simulink model "FOC_Motor_Control"  (R2020b)
settings: Solver=FixedStepAuto  StartTime=0.0  StopTime=10.0  FixedStep=Fixed_Step_Size  RelTol=1e-3
values from neighbouring files (symbols this model uses):
  Angle = 1.0    [Hall_FOC_Data.sldd]
  Angle_offset = 0.1985    [Hall_FOC_Data.sldd]
  atan_table = -1.5690511 -1.5690503 -1.5690495 -1.5690485 -1.5690477 -1.5690469 -1.569046 -1.5690452 -1.5690442 -1.5690434 -1.5690426 -1.5690417 -1.5690409 -1.5690399 -1.5690391 -1.5690383 -1.5690374 -1.5690365 -1.5690356 -1.5690348 -1.5690339 -1.569033 -1.5690322 -1.5690314 -1.5690304 -1.5690296 -1.5690287 -1.5690278 -1.5690269 -1.5690261 -1.5690252 -1.5690243 -1.5690234 -1.5690225 -1.5690217 -1.5690207 -1.569    [Hall_FOC_Data.sldd]
  Cosine_table = 1.0 0.99999529 0.99999058 0.99998587 0.99998116 0.99996704 0.99995291 0.99993885 0.99992472 0.99990118 0.99987763 0.99985409 0.9998306 0.99979764 0.99976468 0.99973178 0.99969882 0.99965644 0.99961412 0.99957174 0.99952942 0.99947762 0.99942589 0.99937415 0.99932235 0.9992612 0.99920005 0.99913889 0.99907768 0.99900717 0.99893659 0.99886602 0.99879545 0.99871546 0.99863547 0.99855554 0.99847555 0.    [Hall_FOC_Data.sldd]
  Dead_Com_Enable = 0.0    [Hall_FOC_Data.sldd]
  Dead_Time = 0.0    [Hall_FOC_Data.sldd]
  FF_Enable = 0.0    [Hall_FOC_Data.sldd]
  Flux = 0.0260812    [Hall_FOC_Data.sldd]
  FluxWeak_Enable = 0.0    [Hall_FOC_Data.sldd]
  FluxWeak_Idref_max = 0.0    [Hall_FOC_Data.sldd]
  FluxWeak_Idref_min = -200.0    [Hall_FOC_Data.sldd]
  FluxWeak_Ki = 50.0    [Hall_FOC_Data.sldd]
  FluxWeak_Kp = 1.2    [Hall_FOC_Data.sldd]
  HaLL_AngleShift = -0.25    [Hall_FOC_Data.sldd]
  HaLL_Sector1 = 5.236    [Hall_FOC_Data.sldd]
  HaLL_Sector2 = 1.0472    [Hall_FOC_Data.sldd]
  HaLL_Sector3 = 0.0    [Hall_FOC_Data.sldd]
  HaLL_Sector4 = 3.1415    [Hall_FOC_Data.sldd]
  HaLL_Sector5 = 4.1888    [Hall_FOC_Data.sldd]
  HaLL_Sector6 = 2.0944    [Hall_FOC_Data.sldd]
  HaLL_Timer_T = 1.0E-5    [Hall_FOC_Data.sldd]
  Harmonic_Com_Enable = 0.0    [Hall_FOC_Data.sldd]
  Harmonic_Id5th_Ki = 32.0    [Hall_FOC_Data.sldd]
  Harmonic_Id5th_Kp = 1.2    [Hall_FOC_Data.sldd]
  Harmonic_Id5th_Max = 60.0    [Hall_FOC_Data.sldd]
  Harmonic_Id5th_Min = -60.0    [Hall_FOC_Data.sldd]
  Harmonic_Id7th_Ki = 24.0    [Hall_FOC_Data.sldd]
  Harmonic_Id7th_Kp = 0.8    [Hall_FOC_Data.sldd]
  Harmonic_Id7th_Max = 60.0    [Hall_FOC_Data.sldd]
  Harmonic_Id7th_Min = -60.0    [Hall_FOC_Data.sldd]
  Harmonic_Iq5th_Ki = 32.0    [Hall_FOC_Data.sldd]
  Harmonic_Iq5th_Kp = 1.2    [Hall_FOC_Data.sldd]
  Harmonic_Iq5th_Max = 60.0    [Hall_FOC_Data.sldd]
  Harmonic_Iq5th_Min = -60.0    [Hall_FOC_Data.sldd]
  Harmonic_Iq7th_Ki = 24.0    [Hall_FOC_Data.sldd]
  Harmonic_Iq7th_Kp = 0.8    [Hall_FOC_Data.sldd]
  Harmonic_Iq7th_Max = 60.0    [Hall_FOC_Data.sldd]
  Harmonic_Iq7th_Min = -60.0    [Hall_FOC_Data.sldd]
  ID_Ki = 0.8    [Hall_FOC_Data.sldd]
  ID_Kp = 3.2    [Hall_FOC_Data.sldd]
  IQ_Ki = 0.32    [Hall_FOC_Data.sldd]
  IQ_Kp = 3.3    [Hall_FOC_Data.sldd]
  LADRC_b0 = 80000.0    [Hall_FOC_Data.sldd]
  LADRC_Omega_c = 80.0    [Hall_FOC_Data.sldd]
  Ld = 0.004    [Hall_FOC_Data.sldd]
  Lq = 0.0042    [Hall_FOC_Data.sldd]
  MTPA_id_table = 0.22889 0.23462678 0.23770036 0.2381243 0.23591207 0.23107713 0.2236329 0.21359272 0.20096992 0.18577772 0.16802935 0.14773798 0.12491672 0.099578641 0.071736768 0.041404068 0.0085934745 -0.026682133 -0.064409919 -0.10457709 -0.14717092 -0.1921787 -0.2395878 -0.28938559 -0.34155953 -0.39609709 -0.45298585 -0.51221335 -0.57376724 -0.63763517 -0.70380485 -0.77226412 -0.84300071 -0.91600245 -0.991257    [Hall_FOC_Data.sldd]
  MTPA_iq_table = -1.0417 -0.16083497 0.71926296 1.5985928 2.4771533 3.3549435 4.2319627 5.1082091 5.9836826 6.8583813 7.732305 8.6054525 9.4778223 10.349415 11.220228 12.090261 12.959513 13.827983 14.69567 15.562573 16.428694 17.294027 18.158575 19.022335 19.885307 20.747492 21.608887 22.469492 23.329306 24.188328 25.046556 25.903992 26.760633 27.616482 28.471533 29.325788 30.179247 31.031908 31.883772 32.734837 3    [Hall_FOC_Data.sldd]
  MTPA_Te_Max = 800.0    [Hall_FOC_Data.sldd]
  MTPA_Te_Min = 0.0    [Hall_FOC_Data.sldd]
  Over_modulation = 0.0    [Hall_FOC_Data.sldd]
  Pole_Pairs = 2.0    [Hall_FOC_Data.sldd]
  PWM_Frequency = 10000.0    [Hall_FOC_Data.sldd]
  R = 0.4    [Hall_FOC_Data.sldd]
  Sine_table = 0.0 0.0015339879 0.0030679768 0.0046019657 0.0061359555 0.0076698866 0.0092038177 0.010737749 0.012271681 0.013805497 0.015339312 0.016873131 0.018406944 0.019940587 0.021474229 0.023007872 0.024541514 0.026074925 0.027608337 0.029141748 0.03067516 0.032208283 0.033741407 0.035274528 0.036807653 0.038340431 0.039873205 0.04140598 0.042938754 0.04447113 0.046003502 0.047535874 0.049068246 0.0506001    [Hall_FOC_Data.sldd]
  Speed_Ki = 0.633    [Hall_FOC_Data.sldd]
  Speed_Kp = 0.0267    [Hall_FOC_Data.sldd]
  Speed_PI_OutputMax = 5.0    [Hall_FOC_Data.sldd]
  Speed_PI_OutputMin = -5.0    [Hall_FOC_Data.sldd]
  SpeedFilter_Fn = 0.2    [Hall_FOC_Data.sldd]
  TorqueMode = 0.0    [Hall_FOC_Data.sldd]
undefined symbols (not defined in the file or in its folder): DiscIntNeverNeededParam, inverter, magnitude, SVPWM
libraries: simulink x6, powerlib_extras x4, pid_lib x1
(part 2 of 5)

== system FOC_Motor_Control/Motor_Control/Motor_Control_Function/SYM_State_10ms/LPF1 ==
  u : Inport
  Add : Sum  Inputs=+-
  Add1 : Sum
  Constant1 : Constant  Value=0.005  OutDataTypeStr=single
  Divide1 : Product  Inputs=**
  Unit Delay : UnitDelay  SampleTime=-1  HasFrameUpgradeWarning=on
  y : Outport
  wires:
  Constant1/1 -> Divide1/1
  u/1 -> Add/1
  Add/1 -> Divide1/2
  Divide1/1 -> Add1/1
  Unit Delay/1 -> Add/2, Add1/2
  Add1/1 -> Unit Delay/1, y/1

== system FOC_Motor_Control/Motor_Control/Motor_Control_Function/SYM_State_10ms/Power_Cacl ==
  Id : Inport
  Vd : Inport  Port=2
  Iq : Inport  Port=3
  Vq : Inport  Port=4
  Add : Sum
  Product : Product
  Product1 : Product
  Power : Outport
  wires:
  Id/1 -> Product/1
  Vd/1 -> Product/2
  Iq/1 -> Product1/1
  Vq/1 -> Product1/2
  Product/1 -> Add/1
  Product1/1 -> Add/2
  Add/1 -> Power/1

== system FOC_Motor_Control/Motor_Control/Motor_Control_Function/SYM_State_10ms/Torque_Cacl ==
  Id : Inport
  Iq : Inport  Port=2
  Constant : Constant  Value=3/2  OutDataTypeStr=single
  Constant1 : Constant  Value=Pole_Pairs  OutDataTypeStr=single
  Constant2 : Constant  Value=Flux  OutDataTypeStr=single
  Constant3 : Constant  Value=Ld  OutDataTypeStr=single
  Constant4 : Constant  Value=Lq  OutDataTypeStr=single
  Product{,1..4} (5 alike) : Product
  Subtract : Sum
  Subtract1 : Sum  Inputs=+-
  Torque : Outport
  wires:
  Constant1/1 -> Product/1
  Constant/1 -> Product/2
  Constant2/1 -> Product1/1
  Iq/1 -> Product1/2, Product3/1
  Product1/1 -> Subtract/1
  Constant3/1 -> Subtract1/1
  Constant4/1 -> Subtract1/2
  Subtract1/1 -> Product2/1
  Id/1 -> Product2/2
  Product2/1 -> Product3/2
  Product3/1 -> Subtract/2
  Product/1 -> Product4/1
  Subtract/1 -> Product4/2
  Product4/1 -> Torque/1

== system FOC_Motor_Control/Motor_Control/Motor_Control_Function/Angle_Speed_100us/Resolver_Observer/Angle_calibration ==
  Angle_input : Inport
  Angle_offset : Constant  Value=Angle_offset
  If Action Subsystem1 : Subsystem  TreatAsAtomicUnit=on
  If Action Subsystem2 : Subsystem  TreatAsAtomicUnit=on
  If1 : If  IfExpression=u1 > 6.283185307
  Merge1 : Merge
  Subtract1 : Sum
  Angle_output : Outport
  wires:
  Angle_input/1 -> Subtract1/1
  Merge1/1 -> Angle_output/1
  Angle_offset/1 -> Subtract1/2  "Control_ModeCommand"
  If1/1 -> If Action Subsystem2/Action
  If1/2 -> If Action Subsystem1/Action
  If Action Subsystem2/1(Out1) -> Merge1/1
  Subtract1/1 -> If Action Subsystem1/1(In1), If Action Subsystem2/1(In1), If1/1
  If Action Subsystem1/1(Out1) -> Merge1/2

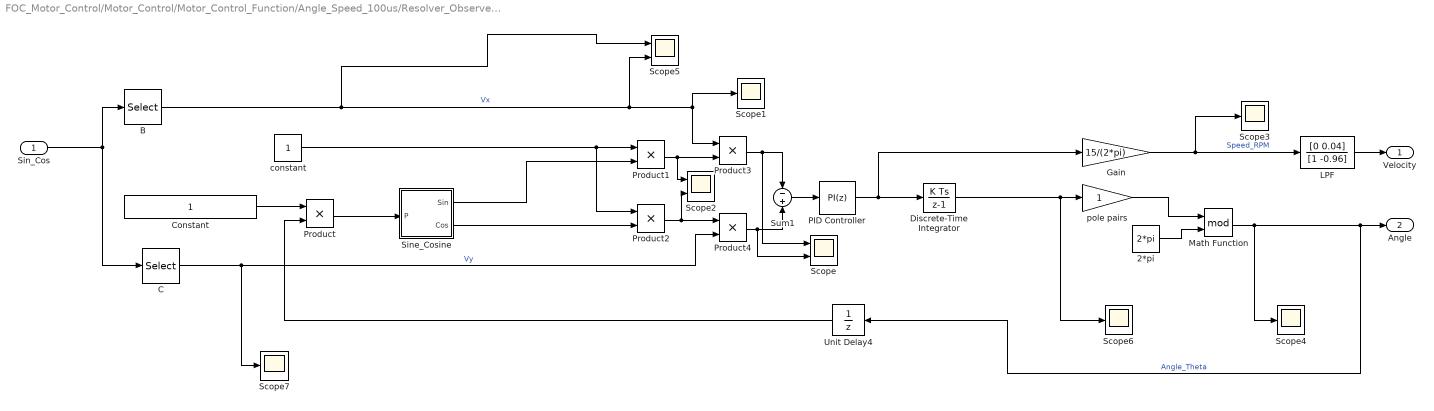
== system FOC_Motor_Control/Motor_Control/Motor_Control_Function/Angle_Speed_100us/Resolver_Observer/Resolver_Angle_cacl ==
  Sin_Cos : Inport
  2*pi : Constant  Value=2*pi  OutDataTypeStr=single  SampleTime=-1
  B : Selector  IndexMode=Zero-based  InputPortWidth=2  IndexOptions=Index vector (dialog)  Indices=0  OutputSizes=1
  C : Selector  IndexMode=Zero-based  InputPortWidth=2  IndexOptions=Index vector (dialog)  Indices=1  OutputSizes=1
  Constant : Constant  OutDataTypeStr=single  SampleTime=-1
  Discrete-Time Integrator : DiscreteIntegrator  SampleTime=-1  ICPrevOutput=DiscIntNeverNeededParam  ICPrevScaledInput=DiscIntNeverNeededParam
  Gain : Gain  Gain=15/(2*pi)
  LPF : DiscreteFilter  Numerator=[0 0.04]  Denominator=[1 -0.96]
  Math Function : Math  Operator=mod  SignedPower=on  SaturateOnIntegerOverflow=on
  PID Controller : pid_lib/PID Controller  Controller=PI  Form=Parallel  TimeDomain=Discrete-time  UseExternalTs=off  SampleTime=-1  IntegratorMethod=Forward Euler  FilterMethod=Forward Euler  ControllerParametersSource=internal  P=141  I=10000  D=0  UseFilter=off  N=100  TunerSelectOption=Transfer Function Based (PID Tuner App)  InitialConditionSource=internal  InitialConditionForIntegrator=0  InitialConditionForFilter=0  DifferentiatorICPrevScaledInput=0  ExternalReset=none  TrackingMode=off  Kt=1  LimitOutput=off  SatLimitsSource=internal  UpperSaturationLimit=inf  LowerSaturationLimit=-inf  LinearizeAsGain=on  AntiWindupMode=none  Kb=1  POutMin=[]  POutMax=[]  IOutMin=[]  IOutMax=[]  DOutMin=[]  DOutMax=[]  NOutMin=[]  NOutMax=[]  SumOutMin=[]  SumOutMax=[]  SaturationOutMin=[]  SaturationOutMax=[]  PParamMin=[]  PParamMax=[]  IParamMin=[]  IParamMax=[]  DParamMin=[]  DParamMax=[]  NParamMin=[]  NParamMax=[]  KbParamMin=[]  KbParamMax=[]  KtParamMin=[]  KtParamMax=[]  KbOutMin=[]  KbOutMax=[]  KtOutMin=[]  KtOutMax=[]  IntegratorOutMin=[]  IntegratorOutMax=[]  FilterOutMin=[]  FilterOutMax=[]  SumI1OutMin=[]  SumI1OutMax=[]  SumI2OutMin=[]  SumI2OutMax=[]  SumI3OutMin=[]  SumI3OutMax=[]  SumI4OutMin=[]  SumI4OutMax=[]  SumDOutMin=[]  SumDOutMax=[]  DifferentiatorOutMin=[]  DifferentiatorOutMax=[]  FilterDiffOutCoefMin=[]  FilterDiffOutCoefMax=[]  ReciprocalOutMin=[]  ReciprocalOutMax=[]  SumDenOutMin=[]  SumDenOutMax=[]  SumNumOutMin=[]  SumNumOutMax=[]  DivideOutMin=[]  DivideOutMax=[]  UdiffTsProdOutMin=[]  UdiffTsProdOutMax=[]  NTsProdOutMin=[]  NTsProdOutMax=[]  UintegralTsProdOutMin=[]  UintegralTsProdOutMax=[]  UngainTsProdOutMin=[]  UngainTsProdOutMax=[]  IntegratorContinuousStateAttributes=''  IntegratorStateMustResolveToSignalObject=off  IntegratorRTWStateStorageClass=Auto  FilterContinuousStateAttributes=''  FilterStateMustResolveToSignalObject=off  FilterRTWStateStorageClass=Auto  ParallelPVariant=InternalParameters  IdealPVariant=Disabled  IVariant=InternalParameters  DVariant=Disabled  IntegratorVariant=Discrete  SatVariant=Disabled  AWVariant=Passthrough  PCopyVariant=Disabled  TRVariant=Disabled  FdbkBlocksVariant=Forward  IdealPFdbkVariant=Disabled  SatFdbkVariant=Disabled  DerivativeFilterVariant=Disabled  NVariant=Disabled  NCopyVariant=Disabled_SignalSpec  FilterICVariant=Disabled  IntegratorICVariant=InternalICs  ExternalResetVariant=Disabled  TRSumVariant=Passthrough  SumFdbkVariant=Disabled  SumVariant=Sum_PI  TsampFilterVariant=InternalTs  TsampNgainVariant=Passthrough  TsampIntegralVariant=Passthrough  ExternalSaturationOutDataTypeStr=Inherit: Same as second input
  Product : Product  OutDataTypeStr=single
  Product{1..4} (4 alike) : Product
  Scope : Scope  NumInputPorts=2
  Scope{1,3..4,6..7} (5 alike) : Scope
  Scope2 : Scope  NumInputPorts=2
  Scope5 : Scope  NumInputPorts=2
  Sine_Cosine : Subsystem  TreatAsAtomicUnit=on
      settings: RTWSystemCode=Nonreusable function  RTWFcnNameOpts=Use subsystem name
  Sum1 : Sum  Inputs=-+
  Unit Delay4 : UnitDelay  SampleTime=-1  HasFrameUpgradeWarning=on
  constant : Constant  OutDataTypeStr=single
  "pole pairs " : Gain  OutDataTypeStr=single
  Velocity : Outport  VectorParamsAs1DForOutWhenUnconnected=off
  Angle : Outport  Port=2  VectorParamsAs1DForOutWhenUnconnected=off
  wires:
  Product2/1 -> Scope2/2, Product4/1
  Product4/1 -> Scope/2, Sum1/2
  Sin_Cos/1 -> C/1, B/1
  Unit Delay4/1 -> Product/2
  Sum1/1 -> PID Controller/1
  Product3/1 -> Scope/1, Sum1/1
  Constant/1 -> Product/1
  constant/1 -> Product2/1, Product1/1
  Product/1 -> Sine_Cosine/1(P)
  Sine_Cosine/1(Sin) -> Product1/2
  Product1/1 -> Scope2/1, Product3/2
  Math Function/1 -> Unit Delay4/1, Angle/1, Scope4/1  "Angle_Theta"
  Gain/1 -> LPF/1, Scope3/1  "Speed_RPM"
  Discrete-Time Integrator/1 -> Scope6/1, "pole pairs "/1
  "pole pairs "/1 -> Math Function/1
  PID Controller/1 -> Discrete-Time Integrator/1, Gain/1
  2*pi/1 -> Math Function/2
  B/1 -> Scope1/1, Product3/1, Scope5/2, Scope5/1  "Vx"
  C/1 -> Product4/2, Scope7/1  "Vy"
  LPF/1 -> Velocity/1
  Sine_Cosine/2(Cos) -> Product2/2

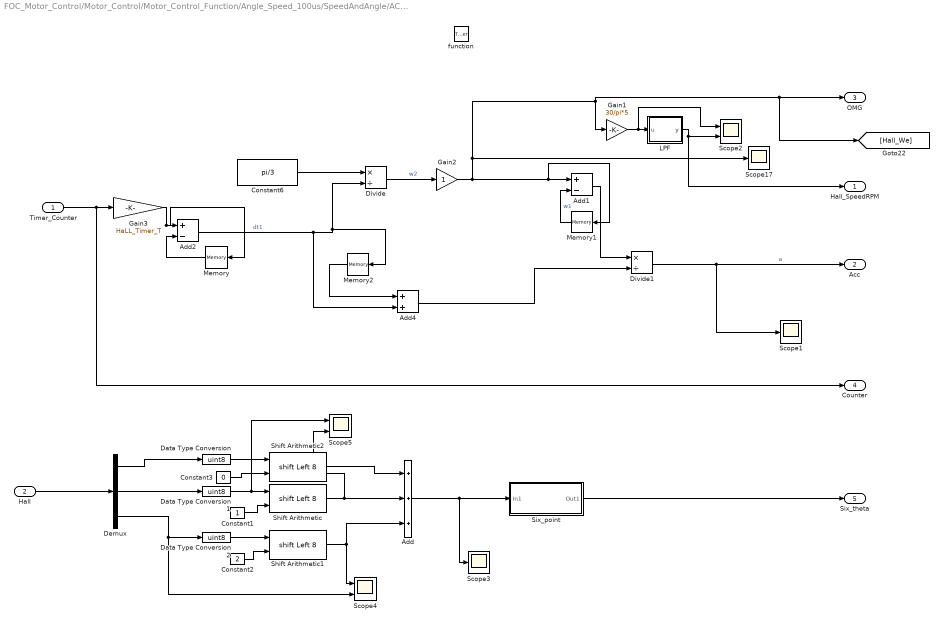
== system FOC_Motor_Control/Motor_Control/Motor_Control_Function/Angle_Speed_100us/SpeedAndAngle/ACC_OMG ==
  Timer_Counter : Inport
  Hall : Inport  Port=2
  function : TriggerPort  TriggerType=either  VariantControl=Variant
  Add : Sum  Inputs=+++
  Add1 : Sum  Inputs=+-
  Add2 : Sum  Inputs=+-
  Add4 : Sum
  Constant1 : Constant  OutDataTypeStr=uint8
  Constant2 : Constant  Value=2  OutDataTypeStr=uint8
  Constant3 : Constant  Value=0  OutDataTypeStr=uint8
  Constant6 : Constant  Value=pi/3  OutDataTypeStr=single
  Data Type Conversion : DataTypeConversion  OutDataTypeStr=uint8
  Data Type Conversion1 : DataTypeConversion  OutDataTypeStr=uint8
  Data Type Conversion2 : DataTypeConversion  OutDataTypeStr=uint8
  Demux : Demux  Outputs=3
  Divide : Product  Inputs=*/
  Divide1 : Product  Inputs=*/
  Gain1 : Gain  Gain=30/pi*5  OutDataTypeStr=Inherit: Same as input  ParamDataTypeStr=Inherit: Same as input
  Gain2 : Gain  OutDataTypeStr=Inherit: Same as input  ParamDataTypeStr=Inherit: Same as input
  Gain3 : Gain  Gain=HaLL_Timer_T
  LPF : Subsystem
  Memory : Memory  InheritSampleTime=on
  Memory1 : Memory  InheritSampleTime=on
  Memory2 : Memory  InheritSampleTime=on
  Scope1 : Scope
  Scope17 : Scope
  Scope2 : Scope  NumInputPorts=2
  Scope3 : Scope
  Scope4 : Scope  NumInputPorts=2
  Scope5 : Scope  NumInputPorts=2
  Shift Arithmetic : ArithShift  BitShiftNumberSource=Input port  BitShiftNumber=8  BitShiftDirection=Left
      settings: InputPortMap=u0,p1
  Shift Arithmetic1 : ArithShift  BitShiftNumberSource=Input port  BitShiftNumber=8  BitShiftDirection=Left
      settings: InputPortMap=u0,p1
  Shift Arithmetic2 : ArithShift  BitShiftNumberSource=Input port  BitShiftNumber=8  BitShiftDirection=Left
      settings: InputPortMap=u0,p1
  Six_point : Subsystem  TreatAsAtomicUnit=on
  Hall_SpeedRPM : Outport
  Acc : Outport  Port=2
  OMG : Outport  Port=3
  Counter : Outport  Port=4
  Six_theta : Outport  Port=5
  wires:
  Timer_Counter/1 -> Counter/1, Gain3/1
  Constant6/1 -> Divide/1
  Divide/1 -> Gain2/1  "w2"
  Memory/1 -> Add2/2
  Add2/1 -> Add4/2, Memory2/1, Divide/2  "dt1"
  Memory1/1 -> Add1/2  "w1"
  Add1/1 -> Divide1/1
  Add4/1 -> Divide1/2
  Divide1/1 -> Acc/1, Scope1/1  "a"
  Gain3/1 -> Memory/1, Add2/1
  Memory2/1 -> Add4/1
  Demux/3 -> Scope4/2, Data Type Conversion2/1
  Data Type Conversion2/1 -> Shift Arithmetic1/1
  Constant2/1 -> Shift Arithmetic1/2
  Constant1/1 -> Shift Arithmetic/2
  Data Type Conversion1/1 -> Scope5/1, Shift Arithmetic/1
  Demux/1 -> Data Type Conversion/1
  Shift Arithmetic/1 -> Add/2, Scope5/2
  Demux/2 -> Data Type Conversion1/1
  Six_point/1(Out1) -> Six_theta/1
  Gain2/1 -> Gain1/1, [Hall_We], OMG/1, Scope17/1, Memory1/1, Add1/1
  Shift Arithmetic1/1 -> Add/3, Scope4/1
  Add/1 -> Scope3/1, Six_point/1(In1)
  Data Type Conversion/1 -> Shift Arithmetic2/1
  Shift Arithmetic2/1 -> Add/1
  Constant3/1 -> Shift Arithmetic2/2
  Hall/1 -> Demux/1
  LPF/1(y) -> Scope2/2, Hall_SpeedRPM/1
  Gain1/1 -> Scope2/1, LPF/1(u)

== system FOC_Motor_Control/Motor_Control/Motor_Control_Function/Angle_Speed_100us/SpeedAndAngle/ADC_IRQ ==
  Counter_ADC_IRQ : Inport
  Acc : Inport  Port=2
  OMG : Inport  Port=3
  Counter_Hall_IRQ : Inport  Port=4
  Six_theta : Inport  Port=5
  Add6 : Sum  Inputs=+-
  Add7 : Sum
  Gain2 : Gain  Gain=HaLL_Timer_T
  Gain3 : Gain  Gain=HaLL_Timer_T
  Gain4 : Gain  Gain=0.5
  Gain5 : Gain
  HallAngle_calibration : Subsystem
      settings: RTWSystemCode=Nonreusable function  RTWFcnNameOpts=Use subsystem name
  Math Function1 : Math  Operator=magnitude^2  SaturateOnIntegerOverflow=on
  Minus2 : Sum
  Product1 : Product
  Product2 : Product
  Hall_Angle : Outport
  wires:
  Gain5/1 -> Minus2/2
  Gain3/1 -> Math Function1/1
  Product2/1 -> Gain4/1
  Counter_Hall_IRQ/1 -> Add6/2
  Gain4/1 -> Minus2/1
  Add6/1 -> Gain3/1, Product1/2
  Math Function1/1 -> Product2/2
  Product1/1 -> Gain2/1
  Gain2/1 -> Gain5/1
  Counter_ADC_IRQ/1 -> Add6/1
  OMG/1 -> Product1/1
  Add7/1 -> HallAngle_calibration/1(Angle_input)
  Minus2/1 -> Add7/1
  Six_theta/1 -> Add7/2
  HallAngle_calibration/1(Angle_output) -> Hall_Angle/1  "SMO_Angle"
  Acc/1 -> Product2/1

== system FOC_Motor_Control/Motor_Control/Motor_Control_Function/Angle_Speed_100us/Speed_Resolver/Speed_cacl ==
  note: Speed_Measured
  position : Inport  OutMin=-4*pi  OutMax=4*pi
      settings: AttributesFormatString="------------------\\nMin =  %<OutMin>\\nMax =  %<OutMax>"
  Constant : Constant  Value=pi/(2^31 -1)/(1/PWM_Frequency)  OutDataTypeStr=single
  Constant1 : Constant  Value=1/Pole_Pairs  OutDataTypeStr=single
  Difference_Wrap : Sum  Inputs=+-  AccumDataTypeStr=int32  OutDataTypeStr=int32
  Difference_to_Single : DataTypeConversion  OutDataTypeStr=single
  Difference_to_Single1 : DataTypeConversion  OutDataTypeStr=int32
  Gain : Gain  Gain=60/(2*pi)
  LPF : Subsystem
  Position_Delay : Delay  DelayLength=1
  Product : Product
  Product1 : Product
  Scale_Input : Gain  Gain=((2^31) - 1)/(4*pi)  ParamDataTypeStr=single  OutDataTypeStr=single
      settings: AttributesFormatString=---------------------------------\n%<Gain>
  Scope : Scope  NumInputPorts=2
  Wrap_To_Pi : Gain  Gain=4  RndMeth=Simplest  OutDataTypeStr=Inherit: Same as input  ParamDataTypeStr=Inherit: Same as input
  Speed_RPM : Outport  VectorParamsAs1DForOutWhenUnconnected=off
  wires:
  position/1 -> Scale_Input/1  "position"
  Difference_to_Single/1 -> Product/2
  Wrap_To_Pi/1 -> Difference_Wrap/1, Position_Delay/1
  Position_Delay/1 -> Difference_Wrap/2
  Scale_Input/1 -> Difference_to_Single1/1
  Difference_Wrap/1 -> Difference_to_Single/1
  Constant/1 -> Product/1
  Constant1/1 -> Product1/1
  Product/1 -> Gain/1  "We"
  Gain/1 -> Product1/2
  Difference_to_Single1/1 -> Wrap_To_Pi/1
  Product1/1 -> Scope/1, LPF/1(u)
  LPF/1(y) -> Scope/2, Speed_RPM/1

== system FOC_Motor_Control/Motor_Control/Motor_Control_Function/Control_Command_2ms/Control_Command_2ms/Speed_PI ==
  Speed_Command : Inport
  Speed_Measured : Inport  Port=2
  Reset : Inport  Port=3
  Action Port : ActionPort  ActionPortLabel=case [ 0 ]:
  SpeedLoop : Subsystem  Commented=on
  Speed_PI : Subsystem
  Iq_ref : Outport  VectorParamsAs1DForOutWhenUnconnected=off
  wires:
  Speed_PI/1(PI_out) -> Iq_ref/1
  Speed_Command/1 -> Speed_PI/1(Ref)
  Reset/1 -> Speed_PI/3(Reset)
  Speed_Measured/1 -> Speed_PI/2(Fdk)

== system FOC_Motor_Control/Motor_Control/Motor_Control_Function/Control_Command_2ms/Control_Command_2ms/Switch Case Action Subsystem ==
  Iq_in : Inport
  Action Port : ActionPort  ActionPortLabel=case [ 1 ]:
  Iq_out : Outport
  wires:
  Iq_in/1 -> Iq_out/1

== system FOC_Motor_Control/Motor_Control/Motor_Control_Function/Control_Command_2ms/Flux_weakening /Subsystem ==
  Reset : Inport
  Vd : Inport  Port=2
  Vq : Inport  Port=3
  Id : Inport  Port=4
  Iq : Inport  Port=5
  Bus_voltage : Inport  Port=6
  Action Port : ActionPort  ActionPortLabel=if(u1 ==1)
  Flux_weak : Subsystem  TreatAsAtomicUnit=on  mask{kp=FluxWeak_Kp, ki=FluxWeak_Ki, Id_max=FluxWeak_Idref_max, Id_min=FluxWeak_Idref_min}
      settings: RTWSystemCode=Nonreusable function  RTWFcnNameOpts=Use subsystem name
  Id_ref : Outport
  Iq_ref : Outport  Port=2
  wires:
  Vd/1 -> Flux_weak/2(Vd)
  Vq/1 -> Flux_weak/3(Vq)
  Id/1 -> Flux_weak/4(id_input)
  Iq/1 -> Flux_weak/5(Iq_input)
  Flux_weak/1(Id_ref) -> Id_ref/1
  Flux_weak/2(iq_ref) -> Iq_ref/1
  Reset/1 -> Flux_weak/1(Reset)
  Bus_voltage/1 -> Flux_weak/6(Bus_voltage)

== system FOC_Motor_Control/Motor_Control/Motor_Control_Function/Control_Command_2ms/Flux_weakening /Subsystem1 ==
  Id : Inport
  Iq : Inport  Port=2
  Action Port : ActionPort  ActionPortLabel=else
  Id_ref : Outport
  Iq_ref : Outport  Port=2
  wires:
  Id/1 -> Id_ref/1
  Iq/1 -> Iq_ref/1

== system FOC_Motor_Control/Motor_Control/Motor_Control_Function/FOC_Control_100us/FOC/Clarke_Transform ==
  Phase_CurrentABC : Inport  PortDimensions=3
  Clark1 : Subsystem  TreatAsAtomicUnit=on
  Scope : Scope  NumInputPorts=2
  IAlpha : Outport  VectorParamsAs1DForOutWhenUnconnected=off
  IBeta : Outport  Port=2  VectorParamsAs1DForOutWhenUnconnected=off
  wires:
  Clark1/1(Ialpha) -> IAlpha/1, Scope/1
  Clark1/2(Ibeta) -> IBeta/1, Scope/2
  Phase_CurrentABC/1 -> Clark1/1(Iabc)

== system FOC_Motor_Control/Motor_Control/Motor_Control_Function/FOC_Control_100us/FOC/DT_Compensation ==
  Enable : Inport
  Ts : Inport  Port=2
  Td : Inport  Port=3
  Udc : Inport  Port=4
  Id : Inport  Port=5
  Iq : Inport  Port=6
  Theta : Inport  Port=7
  DT_Compensation : Subsystem
  Delta_Ualpha : Outport
  Delta_Ubeta : Outport  Port=2
  wires:
  Enable/1 -> DT_Compensation/Enable
  Td/1 -> DT_Compensation/2(Td)
  Ts/1 -> DT_Compensation/1(Ts)
  Udc/1 -> DT_Compensation/3(Udc)
  Id/1 -> DT_Compensation/4(Id)
  Iq/1 -> DT_Compensation/5(Iq)
  Theta/1 -> DT_Compensation/6(Theta)
  DT_Compensation/2(Delta_Ubeta) -> Delta_Ubeta/1
  DT_Compensation/1(Delta_Ualpha) -> Delta_Ualpha/1

== system FOC_Motor_Control/Motor_Control/Motor_Control_Function/FOC_Control_100us/FOC/D_Current_PI ==
  Reset : Inport
  Bus_voltage : Inport  Port=2
  Current_Command : Inport  Port=3
  Current_Measured : Inport  Port=4
  Add2 : Sum  Inputs=|+-
  ID_Control : Subsystem
  Vd_voltage : Outport  VectorParamsAs1DForOutWhenUnconnected=off
  wires:
  Current_Command/1 -> Add2/1
  Current_Measured/1 -> Add2/2
  Add2/1 -> ID_Control/3(Err)  "currentControlError"
  Reset/1 -> ID_Control/1(Reset)
  Bus_voltage/1 -> ID_Control/2(Bus_voltage)
  ID_Control/1(PI_Out) -> Vd_voltage/1

== system FOC_Motor_Control/Motor_Control/Motor_Control_Function/FOC_Control_100us/FOC/FeedForward ==
  note: Vd=id*Rs-we*Lq*iq
  note: Vq=we*Ld*id+iq*Rs+we*flux
  Enable : Inport
  id : Inport  Port=2
  iq : Inport  Port=3
  we : Inport  Port=4
  Subsystem : Subsystem
  Vd : Outport
  Vq : Outport  Port=2
  wires:
  id/1 -> Subsystem/1(id)
  we/1 -> Subsystem/2(iq)
  iq/1 -> Subsystem/3(we)
  Subsystem/1(Vd) -> Vd/1
  Subsystem/2(Vq) -> Vq/1
  Enable/1 -> Subsystem/Enable

== system FOC_Motor_Control/Motor_Control/Motor_Control_Function/FOC_Control_100us/FOC/Har_Compensation ==
  Enable : Inport
  Ialpha : Inport  Port=2
  Ibeta : Inport  Port=3
  We : Inport  Port=4  OutMin=0  OutMax=2*pi
  Theta : Inport  Port=5  OutMin=0  OutMax=2*pi
  Har_Compensation : Subsystem
  Ualfa57 : Outport  VectorParamsAs1DForOutWhenUnconnected=off
  Ubelt57 : Outport  Port=2  VectorParamsAs1DForOutWhenUnconnected=off
  wires:
  Har_Compensation/2(Ubelt57) -> Ubelt57/1
  Har_Compensation/1(Ualfa57) -> Ualfa57/1
  Theta/1 -> Har_Compensation/4(Theta)
  We/1 -> Har_Compensation/3(We)
  Ibeta/1 -> Har_Compensation/2(Ibeta)
  Ialpha/1 -> Har_Compensation/1(Ialpha)
  Enable/1 -> Har_Compensation/Enable

== system FOC_Motor_Control/Motor_Control/Motor_Control_Function/FOC_Control_100us/FOC/Inverse_Park_Transform ==
  D : Inport
  Q : Inport  Port=2
  Sin_Coefficient : Inport  Port=3
  Cos_Coefficient : Inport  Port=4
  Theta : Inport  Port=5
  Add : Sum
  Add1 : Sum  Inputs=+-  OutDataTypeStr=Inherit: Same as first input
  Add2 : Sum  OutDataTypeStr=Inherit: Same as first input
  Add3 : Sum
  Cos_Coefficient1 : InportShadow  Port=4
  Harmonic_injection : Subsystem  Commented=on
  Product{1..4} (4 alike) : Product  RndMeth=Simplest  OutDataTypeStr=Inherit: Same as first input
  Scope : Scope  NumInputPorts=2
  Sin_Coefficient1 : InportShadow  Port=3
  Alpha : Outport  VectorParamsAs1DForOutWhenUnconnected=off
  Beta : Outport  Port=2  VectorParamsAs1DForOutWhenUnconnected=off
  wires:
  Product3/1 -> Add2/1
  Product4/1 -> Add2/2
  Product1/1 -> Add1/1
  Product2/1 -> Add1/2
  Cos_Coefficient1/1 -> Product4/2
  Sin_Coefficient/1 -> Product2/2
  D/1 -> Product3/1, Product1/1
  Q/1 -> Product2/1, Product4/1
  Sin_Coefficient1/1 -> Product3/2
  Cos_Coefficient/1 -> Product1/2
  Add1/1 -> Add/1
  Add/1 -> Alpha/1
  Harmonic_injection/1(Out1) -> Scope/1, Add/2
  Add2/1 -> Add3/2
  Add3/1 -> Beta/1
  Harmonic_injection/2(Out2) -> Scope/2, Add3/1
  Theta/1 -> Harmonic_injection/1(Input)

== system FOC_Motor_Control/Motor_Control/Motor_Control_Function/FOC_Control_100us/FOC/Park_Transform ==
  Alpha : Inport
  Beta : Inport  Port=2
  Sin_Coefficient : Inport  Port=3
  Cos_Coefficient : Inport  Port=4
  Add1 : Sum  OutDataTypeStr=Inherit: Same as first input
  Add2 : Sum  Inputs=-+  OutDataTypeStr=Inherit: Same as first input
  Alpha1 : InportShadow
  Beta1 : InportShadow  Port=2
  Cos_Coefficient1 : InportShadow  Port=4
  Produc3t : Product  RndMeth=Simplest  OutDataTypeStr=Inherit: Same as first input
  Product1 : Product  RndMeth=Simplest  OutDataTypeStr=Inherit: Same as first input
  Product2 : Product  RndMeth=Simplest  OutDataTypeStr=Inherit: Same as first input
  Product4 : Product  RndMeth=Simplest  OutDataTypeStr=Inherit: Same as first input
  Sin_Coefficient1 : InportShadow  Port=3
  D : Outport  VectorParamsAs1DForOutWhenUnconnected=off
  Q : Outport  Port=2  VectorParamsAs1DForOutWhenUnconnected=off
  wires:
  Produc3t/1 -> Add2/1
  Product4/1 -> Add2/2
  Product1/1 -> Add1/1
  Product2/1 -> Add1/2
  Alpha1/1 -> Produc3t/1
  Sin_Coefficient1/1 -> Produc3t/2
  Cos_Coefficient1/1 -> Product4/2
  Beta1/1 -> Product4/1
  Alpha/1 -> Product1/1
  Cos_Coefficient/1 -> Product1/2
  Beta/1 -> Product2/1
  Sin_Coefficient/1 -> Product2/2
  Add1/1 -> D/1
  Add2/1 -> Q/1

== system FOC_Motor_Control/Motor_Control/Motor_Control_Function/FOC_Control_100us/FOC/Q_Current_PI ==
  Reset : Inport
  Bus_voltage : Inport  Port=2
  Current_Command : Inport  Port=3
  Current_Measured : Inport  Port=4
  Add2 : Sum  Inputs=|+-
  IQ_Control : Subsystem
  Vq_voltage : Outport  VectorParamsAs1DForOutWhenUnconnected=off
  wires:
  Current_Command/1 -> Add2/1
  Current_Measured/1 -> Add2/2
  Add2/1 -> IQ_Control/3(Err)  "currentControlError"
  Reset/1 -> IQ_Control/1(Reset)
  Bus_voltage/1 -> IQ_Control/2(Bus_voltage)
  IQ_Control/1(PI_Out) -> Vq_voltage/1

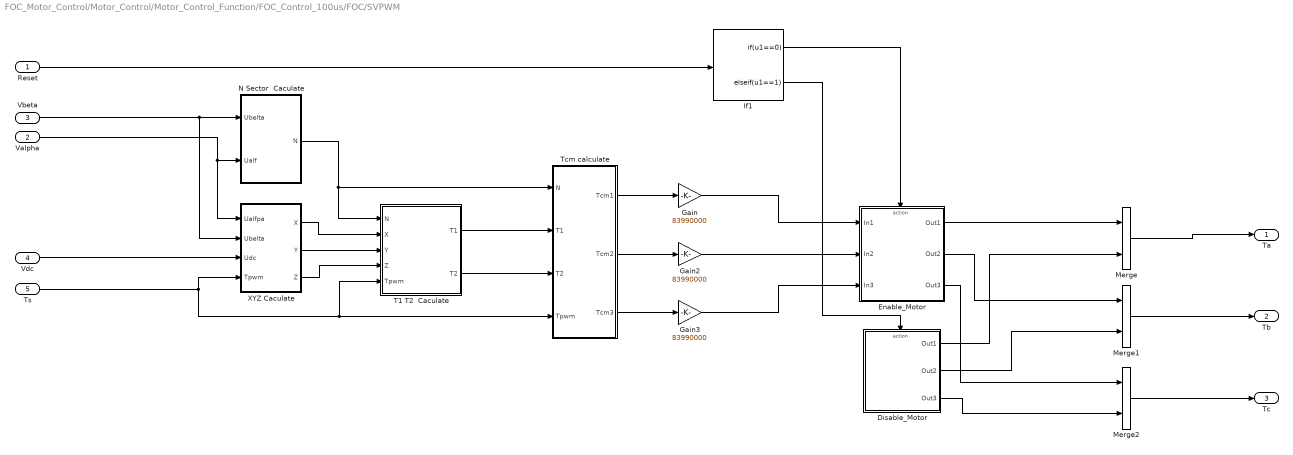
== system FOC_Motor_Control/Motor_Control/Motor_Control_Function/FOC_Control_100us/FOC/SVPWM ==
  Reset : Inport
  Valpha : Inport  Port=2
  Vbeta : Inport  Port=3
  Vdc : Inport  Port=4
  Ts : Inport  Port=5
  Disable_Motor : Subsystem  TreatAsAtomicUnit=on
  Enable_Motor : Subsystem  TreatAsAtomicUnit=on
  Gain : Gain  Gain=83990000
  Gain2 : Gain  Gain=83990000
  Gain3 : Gain  Gain=83990000
  If1 : If  IfExpression=u1==0  ElseIfExpressions=u1==1  ShowElse=off
  Merge : Merge
  Merge1 : Merge
  Merge2 : Merge
  N Sector  Caculate : Subsystem  TreatAsAtomicUnit=on
  T1 T2  Caculate : Subsystem  TreatAsAtomicUnit=on
  Tcm calculate : Subsystem  TreatAsAtomicUnit=on
  XYZ Caculate : Subsystem  TreatAsAtomicUnit=on
  Ta : Outport
  Tb : Outport  Port=2
  Tc : Outport  Port=3
  wires:
  T1 T2  Caculate/2(T2) -> Tcm calculate/3(T2)
  XYZ Caculate/1(X) -> T1 T2  Caculate/2(X)
  N Sector  Caculate/1(N) -> T1 T2  Caculate/1(N), Tcm calculate/1(N)
  Vdc/1 -> XYZ Caculate/3(Udc)
  T1 T2  Caculate/1(T1) -> Tcm calculate/2(T1)
  XYZ Caculate/3(Z) -> T1 T2  Caculate/4(Z)
  XYZ Caculate/2(Y) -> T1 T2  Caculate/3(Y)
  Valpha/1 -> N Sector  Caculate/2(Ualf), XYZ Caculate/1(Ualfpa)
  Vbeta/1 -> N Sector  Caculate/1(Ubelta), XYZ Caculate/2(Ubelta)
  Ts/1 -> T1 T2  Caculate/5(Tpwm), Tcm calculate/4(Tpwm), XYZ Caculate/4(Tpwm)
  Gain/1 -> Enable_Motor/1(In1)
  Gain2/1 -> Enable_Motor/2(In2)
  Reset/1 -> If1/1
  If1/1 -> Enable_Motor/Action
  If1/2 -> Disable_Motor/Action
  Gain3/1 -> Enable_Motor/3(In3)
  Enable_Motor/1(Out1) -> Merge/1
  Disable_Motor/1(Out1) -> Merge/2
  Enable_Motor/2(Out2) -> Merge1/1
  Disable_Motor/2(Out2) -> Merge1/2
  Enable_Motor/3(Out3) -> Merge2/1
  Disable_Motor/3(Out3) -> Merge2/2
  Merge/1 -> Ta/1
  Merge1/1 -> Tb/1
  Merge2/1 -> Tc/1
  Tcm calculate/1(Tcm1) -> Gain/1
  Tcm calculate/2(Tcm2) -> Gain2/1
  Tcm calculate/3(Tcm3) -> Gain3/1

== system FOC_Motor_Control/Motor_Control/Motor_Control_Function/FOC_Control_100us/FOC/Sine_Cosine ==
  note: Sine Cosine Coefficients
  P : Inport
  Cosine : Lookup_n-D  NumberOfTableDimensions=1  LookupTableObject=''  BreakpointsForDimension1=[0:2*pi/4095:2*pi]  BreakpointsForDimension1FirstPoint=10  BreakpointsForDimension2FirstPoint=10  BreakpointsForDimension1Spacing=12  BreakpointsForDimension2Spacing=12  IndexSearchMethod=Evenly spaced points  Table=Cosine_table  InterpMethod=Flat  DiagnosticForOutOfRangeInput=Error  InternalRulePriority=Speed  RndMeth=Simplest  InputSameDT=on
  Saturation : Saturate  UpperLimit=2*pi-0.0001  LowerLimit=0+0.0001
  Scope : Scope  NumInputPorts=2
  Sine : Lookup_n-D  NumberOfTableDimensions=1  LookupTableObject=''  BreakpointsForDimension1=[0:2*pi/4095:2*pi]  BreakpointsForDimension1FirstPoint=10  BreakpointsForDimension2FirstPoint=10  BreakpointsForDimension1Spacing=12  BreakpointsForDimension2Spacing=12  IndexSearchMethod=Evenly spaced points  Table=Sine_table  InterpMethod=Flat  DiagnosticForOutOfRangeInput=Error  InternalRulePriority=Speed  RndMeth=Simplest  InputSameDT=on
  Sin : Outport  VectorParamsAs1DForOutWhenUnconnected=off
  Cos : Outport  Port=2  VectorParamsAs1DForOutWhenUnconnected=off
  wires:
  P/1 -> Saturation/1  "position"
  Sine/1 -> Scope/1, Sin/1
  Cosine/1 -> Scope/2, Cos/1
  Saturation/1 -> Cosine/1, Sine/1

== system FOC_Motor_Control/Motor_Control/Motor_Control_Function/Angle_Speed_100us/Resolver_Observer/Angle_calibration/If Action Subsystem1 ==
  In1 : Inport
  Action Port : ActionPort  ActionPortLabel=else
  Out1 : Outport
  wires:
  In1/1 -> Out1/1

== system FOC_Motor_Control/Motor_Control/Motor_Control_Function/Angle_Speed_100us/Resolver_Observer/Angle_calibration/If Action Subsystem2 ==
  In1 : Inport
  Action Port : ActionPort  ActionPortLabel=if(u1 > 6.283185307)
  2pi : Constant  Value=2*pi  OutDataTypeStr=single
  Subtract1 : Sum  Inputs=+-
  Out1 : Outport
  wires:
  In1/1 -> Subtract1/1
  Subtract1/1 -> Out1/1
  2pi/1 -> Subtract1/2
